simulink model "cartPendulumModel"  (R2017b)
settings: Solver=FixedStepAuto  StartTime=0.0  StopTime=T_final  FixedStep=Ts  RelTol=1e-3
values from neighbouring files (symbols this model uses):
  a = (i_a'\F')    [forceTest.m]    (also in initPendulum.m = 0.47089445904; pplane8.m = max(abs(real([a1,a2]))); testScr.m = 9)
  b = max(abs(imag([a1,a2])))    [pplane8.m]    (also in testScr.m = 0.818181818182)
  b_c_c = (3.021 + 2.746)/2    (= 2.8835)    [initPendulum.m]
  b_c_v = (1.937 + 1.422)/2    (= 1.6795)    [initPendulum.m]
  b_p_c = 4e-3    (= 0.004)    [initPendulum.m]
  b_p_v = .4e-3    (= 0.0004)    [initPendulum.m]
  c = m*l    (= 1.4064948)    [initPendulum.m]    (also in pplane8.m = num2str(wmat(j,3)); testScr.m = 0.272727272727)
  d = M+m    (= 9.474)    [initPendulum.m]    (also in pplane8.m = num2str(wmat(j,4)); testScr.m = 29.46)
  e = m*g*l    (= 13.811778936)    [initPendulum.m]
  g = 9.82    [forceTest.m]    (also in initPendulum.m; plotCartPendulumAnimationOde45.m; simSimpleOdeFun.m; simpleOdeFunSample.m)
  k_tan = 250    [initPendulum.m]
  l = 0.3348    [initPendulum.m]    (also in plotCartPendulumAnimationOde45.m = 0.647; pplane8.m = l+1; simSimpleOdeFun.m = 1; simpleOdeFunSample.m = 1)
  M = 5.273    [initPendulum.m]    (also in plotCartPendulumAnimationOde45.m = 10.546; testScr.m = 10)
  m = 4+.100+.075+.026    (= 4.201)    [initPendulum.m]    (also in plotCartPendulumAnimationOde45.m = 0.402; simSimpleOdeFun.m = 1; simpleOdeFunSample.m = 1; testScr.m = 1)
  theta_0 = pi/2    (= 1.57079632679)    [cartPendulumScr.m]    (also in initPendulum.m; plotCartPendulumAnimationOde45.m = 3.14159265359; run_phasePortraits.m = 5.49778714378; simpleOdeFunSample.m)
  w = exp(i*theta)    [pplane8.m]
libraries: vrlib x4, simulink x3
settings Model: Creator=niels  LastModifiedBy=niels
settings SolverCC: AlgebraicLoopSolver=LineSearch
settings DataIOCC: Refine=200
settings CodeAppCC: StateflowObjectComments=on
settings SimscapeCC: SimscapeNormalizeSystem=off

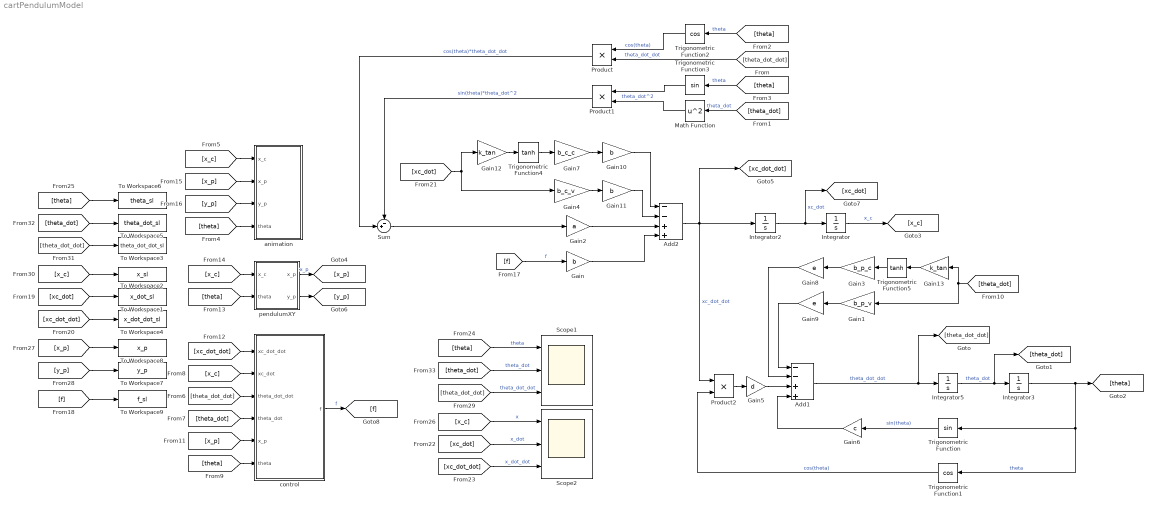
== system cartPendulumModel ==
  Add1 : Sum  Inputs=--++
  Add2 : Sum  Inputs=--++
  Gain : Gain  Gain=b
  Gain1 : Gain  Gain=b_p_v
  Gain10 : Gain  Gain=b
  Gain11 : Gain  Gain=b
  Gain12 : Gain  Gain=k_tan
  Gain13 : Gain  Gain=k_tan
  Gain2 : Gain  Gain=a
  Gain3 : Gain  Gain=b_p_c
  Gain4 : Gain  Gain=b_c_v
  Gain5 : Gain  Gain=d
  Gain6 : Gain  Gain=c
  Gain7 : Gain  Gain=b_c_c
  Gain8 : Gain  Gain=e
  Gain9 : Gain  Gain=e
  Integrator : Integrator
  Integrator2 : Integrator
  Integrator3 : Integrator  InitialCondition=theta_0
  Integrator5 : Integrator
  Math Function : Math  Operator=square  SaturateOnIntegerOverflow=on
  Product : Product
  Product1 : Product
  Product2 : Product
  Scope1 : Scope  NumInputPorts=3
  Scope2 : Scope  NumInputPorts=3
  Sum : Sum  Inputs=-+|
  To Workspace1 : ToWorkspace  VariableName=x_dot_sl  SaveFormat=Timeseries  SampleTime=-1
  To Workspace2 : ToWorkspace  VariableName=x_sl  SaveFormat=Timeseries  SampleTime=-1
  To Workspace3 : ToWorkspace  VariableName=theta_dot_dot_sl  SaveFormat=Timeseries  SampleTime=-1
  To Workspace4 : ToWorkspace  VariableName=x_dot_dot_sl  SaveFormat=Timeseries  SampleTime=-1
  To Workspace5 : ToWorkspace  VariableName=theta_dot_sl  SaveFormat=Timeseries  SampleTime=-1
  To Workspace6 : ToWorkspace  VariableName=theta_sl  SaveFormat=Timeseries  SampleTime=-1
  To Workspace7 : ToWorkspace  VariableName=y_p  SaveFormat=Timeseries  SampleTime=-1
  To Workspace8 : ToWorkspace  VariableName=x_p  SaveFormat=Timeseries  SampleTime=-1
  To Workspace9 : ToWorkspace  VariableName=f_sl  SaveFormat=Timeseries  SampleTime=-1
  Trigonometric Function : Trigonometry
  Trigonometric Function1 : Trigonometry  Operator=cos
  Trigonometric Function2 : Trigonometry  Operator=cos
  Trigonometric Function3 : Trigonometry
  Trigonometric Function4 : Trigonometry  Operator=tanh
  Trigonometric Function5 : Trigonometry  Operator=tanh
  animation : Subsystem
  control : Subsystem
  pendulumXY : Subsystem
  wires:
  Sum/1 -> Gain2/1
  Integrator2/1 -> [xc_dot], Integrator/1  "xc_dot"
  Add2/1 -> Product2/1, Integrator2/1, [xc_dot_dot]  "xc_dot_dot"
  Integrator5/1 -> [theta_dot], Integrator3/1  "theta_dot"
  Integrator/1 -> [x_c]  "x_c"
  Integrator3/1 -> Trigonometric Function/1, Trigonometric Function1/1, [theta]  "theta"
  Math Function/1 -> Product1/2  "theta_dot^2"
  Trigonometric Function/1 -> Gain6/1  "sin(theta)"
  Product1/1 -> Sum/1  "sin(theta)*theta_dot^2"
  Product/1 -> Sum/2  "cos(theta)*theta_dot_dot"
  Gain6/1 -> Add1/4
  Product2/1 -> Gain5/1
  Trigonometric Function1/1 -> Product2/2  "cos(theta)"
  Trigonometric Function2/1 -> Product/1  "cos(theta)"
  Trigonometric Function3/1 -> Product1/1
  pendulumXY/1(x_p) -> [x_p]  "x_p"
  control/1(f) -> [f]  "f"
  [theta_dot_dot] -> Product/2  "theta_dot_dot"
  [theta] -> Trigonometric Function2/1  "theta"
  [theta] -> Trigonometric Function3/1  "theta"
  [theta_dot] -> Math Function/1  "theta_dot"
  [theta] -> animation/4(theta)
  [x_c] -> animation/1(x_c)
  [theta_dot_dot] -> control/3(theta_dot_dot)
  [theta_dot] -> control/4(theta_dot)
  [x_c] -> control/2(xc_dot)
  [theta] -> control/6(theta)
  [x_p] -> control/5(x_p)
  [xc_dot_dot] -> control/1(xc_dot_dot)
  [theta] -> pendulumXY/2(theta)
  [x_c] -> pendulumXY/1(x_c)
  [x_p] -> animation/2(x_p)
  pendulumXY/2(y_p) -> [y_p]
  [y_p] -> animation/3(y_p)
  [f] -> Gain/1  "f"
  [theta] -> To Workspace6/1
  [theta_dot] -> To Workspace5/1
  [theta_dot_dot] -> To Workspace3/1
  [x_c] -> To Workspace2/1
  [xc_dot] -> To Workspace1/1
  [xc_dot_dot] -> To Workspace4/1
  [x_p] -> To Workspace8/1
  [y_p] -> To Workspace7/1
  [f] -> To Workspace9/1
  Gain3/1 -> Gain8/1
  Gain1/1 -> Gain9/1
  [theta_dot] -> Gain13/1, Gain1/1
  Gain9/1 -> Add1/1
  Gain7/1 -> Gain10/1
  Gain4/1 -> Gain11/1
  Gain/1 -> Add2/4
  Add1/1 -> [theta_dot_dot], Integrator5/1  "theta_dot_dot"
  Trigonometric Function4/1 -> Gain7/1
  Trigonometric Function5/1 -> Gain3/1
  Gain13/1 -> Trigonometric Function5/1
  [xc_dot] -> Gain12/1, Gain4/1
  Gain8/1 -> Add1/2
  Gain2/1 -> Add2/3
  Gain11/1 -> Add2/2
  Gain10/1 -> Add2/1
  Gain12/1 -> Trigonometric Function4/1
  Gain5/1 -> Add1/3
  [theta] -> Scope1/1  "theta"
  [x_c] -> Scope2/1  "x"
  [xc_dot] -> Scope2/2  "x_dot"
  [xc_dot_dot] -> Scope2/3  "x_dot_dot"
  [theta_dot_dot] -> Scope1/3  "theta_dot_dot"
  [theta_dot] -> Scope1/2  "theta_dot"

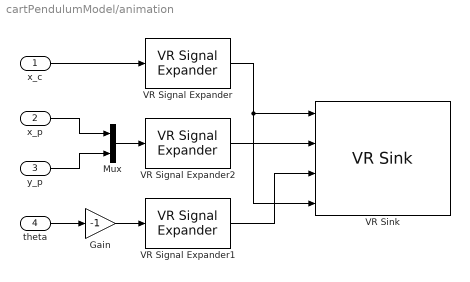
== system cartPendulumModel/animation ==
  x_c : Inport
  x_p : Inport  Port=2
  y_p : Inport  Port=3
  theta : Inport  Port=4
  Gain : Gain  Gain=-1
  Mux : Mux  Inputs=2
  VR Signal Expander : vrlib/VR Signal Expander  outwidth=3  outidx=[1]
      settings: SourceProductName=Simulink 3D Animation  SourceProductBaseCode=VR
  VR Signal Expander1 : vrlib/VR Signal Expander  outwidth=4  outidx=[4]
      settings: SourceProductName=Simulink 3D Animation  SourceProductBaseCode=VR
  VR Signal Expander2 : vrlib/VR Signal Expander  outwidth=3  outidx=[1 2]
      settings: SourceProductName=Simulink 3D Animation  SourceProductBaseCode=VR
  VR Sink : vrlib/VR Sink  InstantiateOnLoad=on  SampleTime=0.01  ViewEnable=on  RemoteChange=off  RemoteView=off  FieldsWritten=cart.translation.3.1.1.double#pendulumMass.translation.3.1.1.double#rod.rotation.4.1.1.double#rod.translation.3.1.1.double  WorldFileName=cartPendulum3D  AutoView=off  VideoDimensions=[]  AllowVariableSize=off
      settings: SourceProductBaseCode=VR
  wires:
  y_p/1 -> Mux/2
  x_c/1 -> VR Signal Expander/1
  x_p/1 -> Mux/1
  theta/1 -> Gain/1
  Mux/1 -> VR Signal Expander2/1
  VR Signal Expander1/1 -> VR Sink/3
  VR Signal Expander/1 -> VR Sink/4, VR Sink/1
  VR Signal Expander2/1 -> VR Sink/2
  Gain/1 -> VR Signal Expander1/1

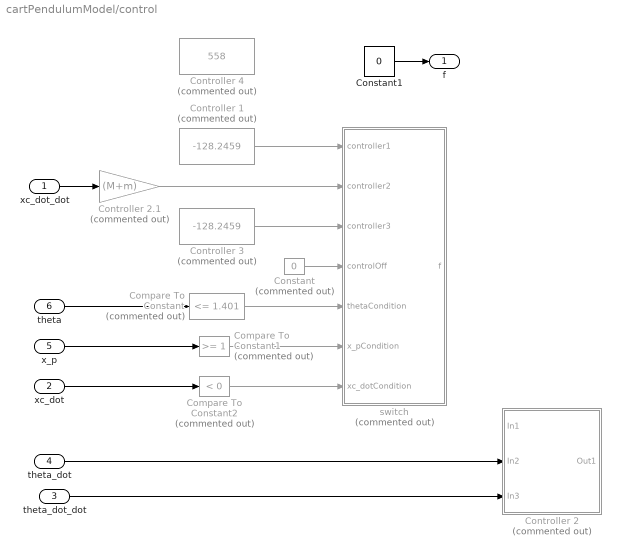
== system cartPendulumModel/control ==
  xc_dot_dot : Inport
  xc_dot : Inport  Port=2
  theta_dot_dot : Inport  Port=3
  theta_dot : Inport  Port=4
  x_p : Inport  Port=5
  theta : Inport  Port=6
  Compare To Constant : simulink/Logic and Bit Operations/Compare To Constant  Commented=on  relop=<=  const=1.401  OutDataTypeStr=boolean
  Compare To Constant1 : simulink/Logic and Bit Operations/Compare To Constant  Commented=on  relop=>=  const=1  OutDataTypeStr=boolean
  Compare To Constant2 : simulink/Logic and Bit Operations/Compare To Constant  Commented=on  relop=<  const=0  OutDataTypeStr=boolean
  Constant : Constant  Commented=on  Value=0
  Constant1 : Constant  Value=0
  Controller 1 : Constant  Commented=on  Value=-128.2459
  Controller 2 : Subsystem  Commented=on
  Controller 2.1 : Gain  Commented=on  Gain=(M+m)
  Controller 3 : Constant  Commented=on  Value=-128.2459
  Controller 4 : Constant  Commented=on  Value=558
  switch : Subsystem  Commented=on
  f : Outport
  wires:
  theta_dot/1 -> Controller 2/2(In2)
  theta/1 -> Compare To Constant/1
  theta_dot_dot/1 -> Controller 2/3(In3)
  x_p/1 -> Compare To Constant1/1
  xc_dot/1 -> Compare To Constant2/1
  xc_dot_dot/1 -> Controller 2.1/1
  Compare To Constant1/1 -> switch/6(x_pCondition)
  Compare To Constant/1 -> switch/5(thetaCondition)
  Controller 1/1 -> switch/1(controller1)
  Controller 3/1 -> switch/3(controller3)
  Compare To Constant2/1 -> switch/7(xc_dotCondition)
  Constant/1 -> switch/4(controlOff)
  Controller 2.1/1 -> switch/2(controller2)
  Constant1/1 -> f/1

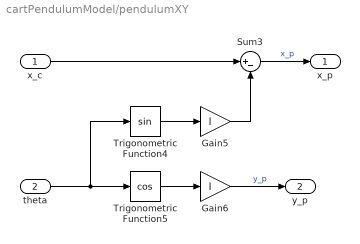
== system cartPendulumModel/pendulumXY ==
  x_c : Inport
  theta : Inport  Port=2
  Gain5 : Gain  Gain=l
  Gain6 : Gain  Gain=l
  Sum3 : Sum  Inputs=|+-
  Trigonometric Function4 : Trigonometry
  Trigonometric Function5 : Trigonometry  Operator=cos
  x_p : Outport
  y_p : Outport  Port=2
  wires:
  x_c/1 -> Sum3/1
  theta/1 -> Trigonometric Function4/1, Trigonometric Function5/1
  Trigonometric Function4/1 -> Gain5/1
  Trigonometric Function5/1 -> Gain6/1
  Gain5/1 -> Sum3/2
  Sum3/1 -> x_p/1  "x_p"
  Gain6/1 -> y_p/1  "y_p"

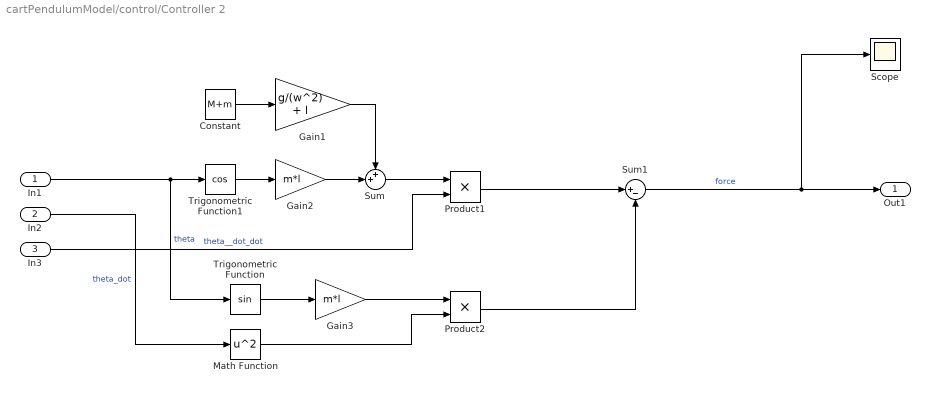
== system cartPendulumModel/control/Controller 2 ==
  In1 : Inport
  In2 : Inport  Port=2
  In3 : Inport  Port=3
  Constant : Constant  Value=M+m
  Gain1 : Gain  Gain=g/(w^2) + l
  Gain2 : Gain  Gain=m*l
  Gain3 : Gain  Gain=m*l
  Math Function : Math  Operator=square  SaturateOnIntegerOverflow=on
  Product1 : Product
  Product2 : Product
  Scope : Scope
  Sum : Sum  Inputs=++|
  Sum1 : Sum  Inputs=|+-
  Trigonometric Function : Trigonometry
  Trigonometric Function1 : Trigonometry  Operator=cos
  Out1 : Outport
  wires:
  In3/1 -> Product1/2  "theta__dot_dot"
  In1/1 -> Trigonometric Function/1, Trigonometric Function1/1  "theta"
  Trigonometric Function1/1 -> Gain2/1
  Gain2/1 -> Sum/2
  Constant/1 -> Gain1/1
  Gain1/1 -> Sum/1
  Sum/1 -> Product1/1
  In2/1 -> Math Function/1  "theta_dot"
  Trigonometric Function/1 -> Gain3/1
  Gain3/1 -> Product2/1
  Math Function/1 -> Product2/2
  Product2/1 -> Sum1/2
  Sum1/1 -> Out1/1, Scope/1  "force"
  Product1/1 -> Sum1/1

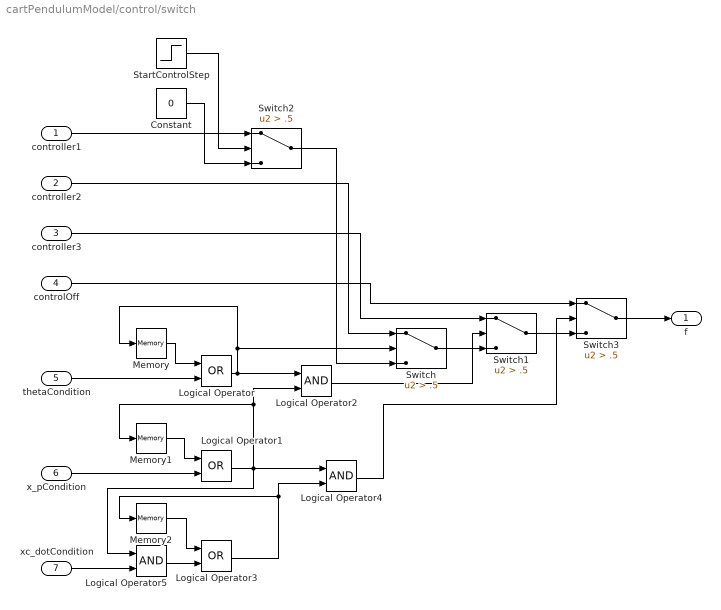
== system cartPendulumModel/control/switch ==
  controller1 : Inport
  controller2 : Inport  Port=2
  controller3 : Inport  Port=3
  controlOff : Inport  Port=4
  thetaCondition : Inport  Port=5
  x_pCondition : Inport  Port=6
  xc_dotCondition : Inport  Port=7
  Constant : Constant  Value=0
  Logical Operator : Logic  Operator=OR  AllPortsSameDT=off  OutDataTypeStr=boolean
  Logical Operator1 : Logic  Operator=OR  AllPortsSameDT=off  OutDataTypeStr=boolean
  Logical Operator2 : Logic  AllPortsSameDT=off  OutDataTypeStr=boolean
  Logical Operator3 : Logic  Operator=OR  AllPortsSameDT=off  OutDataTypeStr=boolean
  Logical Operator4 : Logic  AllPortsSameDT=off  OutDataTypeStr=boolean
  Logical Operator5 : Logic  AllPortsSameDT=off  OutDataTypeStr=boolean
  Memory : Memory
  Memory1 : Memory
  Memory2 : Memory
  StartControlStep : Step  Time=0.0001  SampleTime=0
  Switch{,1..3} (4 alike) : Switch  Criteria=u2 > Threshold  Threshold=.5
  f : Outport
  wires:
  thetaCondition/1 -> Logical Operator/2
  Memory/1 -> Logical Operator/1
  Switch/1 -> Switch1/3
  controller3/1 -> Switch1/1
  Memory1/1 -> Logical Operator1/1
  x_pCondition/1 -> Logical Operator1/2
  Logical Operator1/1 -> Logical Operator5/1, Logical Operator4/1, Logical Operator2/2, Memory1/1
  Logical Operator2/1 -> Switch1/2
  controller2/1 -> Switch/1
  Logical Operator/1 -> Memory/1, Switch/2, Logical Operator2/1
  StartControlStep/1 -> Switch2/2
  Constant/1 -> Switch2/3
  controller1/1 -> Switch2/1
  Switch2/1 -> Switch/3
  Logical Operator3/1 -> Logical Operator4/2, Memory2/1
  Memory2/1 -> Logical Operator3/1
  Switch1/1 -> Switch3/3
  Switch3/1 -> f/1
  controlOff/1 -> Switch3/1
  Logical Operator4/1 -> Switch3/2
  Logical Operator5/1 -> Logical Operator3/2
  xc_dotCondition/1 -> Logical Operator5/2
